simulink model "Model"  (R2025a)
settings: Solver=FixedStepAuto  StartTime=0.0  StopTime=10.0  RelTol=1e-3
values from neighbouring files (symbols this model uses):
  robot = rigidBodyTree('DataFormat','row')    [RigidBodyModel.m]    (also in RigidBodyRobot.m; RigidBodyRobot2.m = rigidBodyTree('DataFormat','row','MaxNumBodies',4))
libraries: robotmaniplib x1
settings Model: Creator=Korisnik  LastModifiedBy=Korisnik

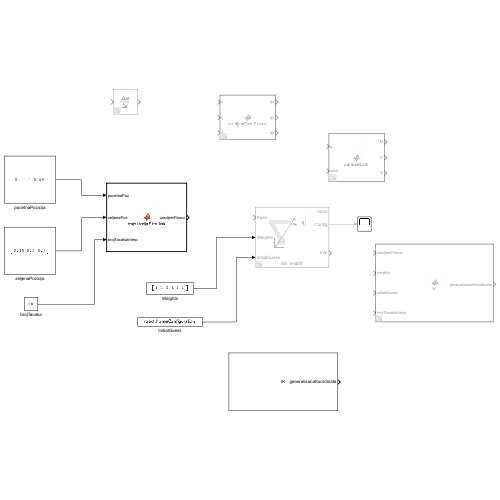
[thumbnail: Simulink's stored preview of the top-level diagram]
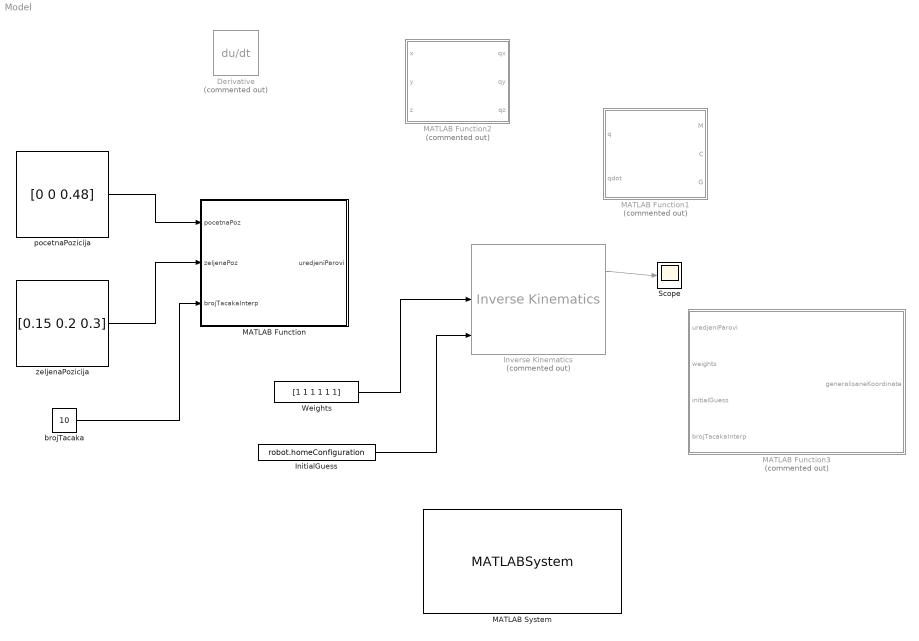
== system Model ==
  Derivative : Derivative  Commented=on
  InitialGuess : Constant  Value=robot.homeConfiguration
  Inverse Kinematics : robotmaniplib/Inverse Kinematics  Commented=on  RigidBodyTree=robot  EndEffector=endEff  ShowInfo=on  SolverName=BFGS Gradient Projection  EnforceJointLimits=on  MaxIterations=1500  MaxTime=10  GradientTolerance=1e-7  SolutionTolerance=1e-6  StepTolerance=1e-14  ConstraintTolerance=1e-6  ErrorChangeTolerance=1e-12  UseErrorDamping=on  DampingBias=0.0025  SimulateUsing=Interpreted execution
  MATLAB Function : MATLAB Function  TreatAsAtomicUnit=on
  MATLAB Function1 : MATLAB Function  Commented=on  TreatAsAtomicUnit=on
  MATLAB Function2 : MATLAB Function  Commented=on  TreatAsAtomicUnit=on
  MATLAB Function3 : MATLAB Function  Commented=on  TreatAsAtomicUnit=on
  MATLAB System : MATLABSystem  System=IK  brojTacakaInterp=[10]  zeljeniPolozaj=[0.1 0.2 0.3]  pocetniPolozaj=[0 0 0.48]  SimulateUsing=Code generation
      mask Type: IK
  Scope : Scope
  Weights : Constant  Value=[1 1 1 1 1 1]
  brojTacaka : Constant  Value=10
  pocetnaPozicija : Constant  Value=[0 0 0.48]
  zeljenaPozicija : Constant  Value=[0.15 0.2 0.3]
  wires:
  pocetnaPozicija/1 -> MATLAB Function/1(pocetnaPoz)
  zeljenaPozicija/1 -> MATLAB Function/2(zeljenaPoz)
  brojTacaka/1 -> MATLAB Function/3(brojTacakaInterp)
  Weights/1 -> Inverse Kinematics/2
  InitialGuess/1 -> Inverse Kinematics/3
  Inverse Kinematics/1 -> Scope/1

== matlab function Model/MATLAB Function1 ==
  data: q input; M output; C output; G output; qdot input
function [M, C, G] = parametriDif(q, qdot)

M = massMatrix(robot, q);
C = velocityProductMatrix(robot, q, qdot);
G = gravityTorque(robot, q);

== matlab function Model/MATLAB Function ==
  data: pocetnaPoz input; uredjeniParovi output; zeljenaPoz input; brojTacakaInterp input
function uredjeniParovi  = trajektorijaSimulink(pocetnaPoz,zeljenaPoz, brojTacakaInterp)
%PRAVLJENJE_TRAJEKTORIJE
%   Za zadati pocetni i krajnji polozaj daje putanje za x, y, z sa n tacaka
%   izmedju
uredjeniParovi = zeros(brojTacakaInterp, 3);
t = [0 1];
tq = linspace(0, 1, brojTacakaInterp);
xPutanja = interp1(t, [pocetnaPoz(1), zeljenaPoz(1)], tq, 'spline');
yPutanja = interp1(t, [pocetnaPoz(2), zeljenaPoz(2)], tq, 'spline');
zPutanja = interp1(t, [pocetnaPoz(3), zeljenaPoz(3)], tq, 'spline');
for i = 1:brojTacakaInterp
    uredjeniParovi(i, :) = [xPutanja(i), yPutanja(i), zPutanja(i)];
end


end

== matlab function Model/MATLAB Function2 ==
  data: qx output; qy output; x input; y input; z input; qz output
function [qx, qy, qz] = uredjeniTrenParovi(x, y, z)
    
for i = 1:10
    qx = x(i);
    qy = y(i);
    qz = z(i);
end

== matlab function Model/MATLAB Function3 ==
  data: uredjeniParovi input; generalisaneKoordinate output; weights input; initialGuess input; brojTacakaInterp input
function generalisaneKoordinate = IK(uredjeniParovi, weights, initialGuess, brojTacakaInterp)

generalisaneKoordinate = zeros(brojTacakaInterp, 4);

ik = inverseKinematics('RigidBodyTree',robot, 'SolverAlgorithm','LevenbergMarquardt');

for i = 1:brojTacakaInterp
    trenutniPolozaj = uredjeniParovi(i, :);
    transformacionaMatrica = trvec2tform(trenutniPolozaj);

    [generalisanaKoordinata, status] = ik('endEff', transformMatrica, weights, initialGuess);
    generalisaneKoordinate(i, :) = generalisanaKoordinata;
    initialGuess = generalisanaKoordinata;
    %Provera da li je ovaj polozaj moguce postici
    if noviPolozaj(2) < min(lakat.PositionLimits) && noviPolozaj(2) > max(lakat.PositionLimits)
        disp('Položaj nije moguće postići.\n');
    end
    if noviPolozaj(3) < min(zglobSake.PositionLimits) && noviPolozaj(4) > max(zglobSake.PositionLimits)
        disp('Položaj nije moguće postići.\n');
    end
    
end



end
